simulink model "simModel2020"  (R2023b)
settings: Solver=ode4  StartTime=0  StopTime=360  FixedStep=0.01  RelTol=1e-3
values from neighbouring files (symbols this model uses):
  B747 =     [B747.mat]
undefined symbols (not defined in the file or in its folder): airport, APP, control, Curise, Earth, env, ft, m, navData, navParam, Newton, plotTrack, Raphson, s, TakeOff, WGS84
libraries: aerolibconvert2 x18, simulink x15, sharedtransform x4, aerolibfltsims x3, aerolibatmos2 x2, shared6dof x2, aerolibasang x2, dspsrcs4 x2, aerolibwind2 x2, aerolibanimutils x1, aerolibpropulsion2 x1, aerolibtransform2 x1
(part 3 of 6)

== system simModel2020/AutoPilot/InnerLoopAutopilot/Latitudinal Channel维度通道/Yaw Select/Filter1 ==
  x : Inport
  SW_x(k-1) : Inport  Port=2
  time : Inport  Port=3
  Constant : Constant  SampleTime=-1
  Data Type Conversion : DataTypeConversion  SaturateOnIntegerOverflow=off  RndMeth=Floor
  Detect Change : simulink/Logic and Bit Operations/Detect Change  vinit=0  OutDataTypeStr=boolean
  Gain : Gain  Gain=0.5
  Math Function : Math  SignedPower=on
  Product : Product
  Product1 : Product
  Subsystem : Subsystem
      mask Display: disp('S/H')
  Sum : Sum  Inputs=|+-
  Sum1 : Sum  Inputs=|++
  Sum2 : Sum  Inputs=+-|
  y : Outport
  wires:
  Product/1 -> Sum1/2
  SW_x(k-1)/1 -> Product/2
  Product1/1 -> Sum1/1
  x/1 -> Product1/1
  Sum1/1 -> Data Type Conversion/1
  time/1 -> Subsystem/1(In), Sum2/2
  Subsystem/1(" ") -> Sum2/1
  Sum2/1 -> Gain/1
  Gain/1 -> Math Function/1
  Math Function/1 -> Product/1, Sum/2
  Sum/1 -> Product1/2
  Data Type Conversion/1 -> y/1
  Constant/1 -> Sum/1, Detect Change/1
  Detect Change/1 -> Subsystem/Enable

== system simModel2020/AutoPilot/InnerLoopAutopilot/Longitudinal Channel经度通道/AutoThrottle/AT Mode = 0,Recycle ==
  dT(k-1) : Inport
  time : Inport  Port=2
  Action Port : ActionPort  InitializeStates=reset  ActionPortLabel=case [ 0 ]:
  Constant : Constant  Value=0.2
  Constant1 : Constant  Value=0
  Constant2 : Constant  Value=-0.2
  Filter1 : Subsystem
  Rate Limiter Dynamic with External IC and Autoreset for Change in IC : Subsystem
      mask Display:
      | plot([0.15 0.95],[.5 .5],[.5 .5],[0.05 0.95],0.05+0.9*[.2 .8],0.05+0.9*[0 1]);
      | port_label('output',1,'Y');
      | port_label('input',1,'up');
      | port_label('input',2,'u');
      | port_label('input',3,'Lo');
      | port_label('input',4,'IC');
  dT : Outport
  wires:
  dT(k-1)/1 -> Rate Limiter Dynamic with External IC and Autoreset for Change in IC/4(IC), Filter1/2(SW_x(k-1))
  Constant1/1 -> Filter1/1(x)
  time/1 -> Filter1/3(time)
  Rate Limiter Dynamic with External IC and Autoreset for Change in IC/1(Y) -> dT/1  "y"
  Filter1/1(y) -> Rate Limiter Dynamic with External IC and Autoreset for Change in IC/2(u)
  Constant/1 -> Rate Limiter Dynamic with External IC and Autoreset for Change in IC/1(up)
  Constant2/1 -> Rate Limiter Dynamic with External IC and Autoreset for Change in IC/3(lo)

== system simModel2020/AutoPilot/InnerLoopAutopilot/Longitudinal Channel经度通道/AutoThrottle/AT Mode = 2,MCP Speed ==
  <U_c> : Inport
  N1 : Inport  Port=2
  <ias> : Inport  Port=3
  dT(k-1) : Inport  Port=4
  time : Inport  Port=5
  Action Port : ActionPort  InitializeStates=reset  ActionPortLabel=case [ 2 ]:
  Add : Sum  Inputs=+-
  Filter1 : Subsystem
  Gain : Gain  Gain=10
  Mux : Mux  Inputs=2
  N1_Control : Subsystem
  Saturation1 : Saturate  UpperLimit=110  LowerLimit=0
  Scope : Scope
  Sum : Sum  Inputs=++|
  sat_integration : Subsystem
  dT : Outport
  wires:
  Gain/1 -> Sum/1
  dT(k-1)/1 -> Filter1/2(SW_x(k-1))
  Filter1/1(y) -> dT/1
  Add/1 -> sat_integration/1(err), Gain/1
  Sum/1 -> Saturation1/1
  N1_Control/1(dT) -> Filter1/1(x)
  N1/1 -> N1_Control/2(N1)
  Saturation1/1 -> N1_Control/1(N1_Cmd)
  sat_integration/1(int_err) -> Sum/2
  time/1 -> Filter1/3(time)
  <ias>/1 -> Mux/2, Add/2
  <U_c>/1 -> Mux/1, Add/1
  Mux/1 -> Scope/1

== system simModel2020/AutoPilot/InnerLoopAutopilot/Longitudinal Channel经度通道/AutoThrottle/AT Mode = 3,Throttle Control ==
  N1_Cmd : Inport
  N1 : Inport  Port=2
  dT(k-1) : Inport  Port=3
  time : Inport  Port=4
  Action Port : ActionPort  InitializeStates=reset  ActionPortLabel=case [ 3 ]:
  Add1 : Sum  Inputs=+-
  Derivative : Derivative
  Filter1 : Subsystem
  Gain : Gain  Gain=0.01
  Gain2 : Gain  Gain=0.02
  Integrator : Integrator
  Mux : Mux  Inputs=2
  Scope : Scope
  Sum : Sum  Inputs=++|
  Throttle Limit3 : Saturate  UpperLimit=0.2  LowerLimit=-0.2
      settings: AttributesFormatString="[%<LowerLimit>  %<UpperLimit>]"
  dT : Outport
  wires:
  Add1/1 -> Gain/1, Derivative/1
  dT(k-1)/1 -> Filter1/2(SW_x(k-1))
  Integrator/1 -> Filter1/1(x)
  Throttle Limit3/1 -> Integrator/1
  Derivative/1 -> Gain2/1
  Sum/1 -> Throttle Limit3/1
  Gain/1 -> Sum/2
  Gain2/1 -> Sum/1
  time/1 -> Filter1/3(time)
  N1/1 -> Mux/2, Add1/2
  N1_Cmd/1 -> Mux/1, Add1/1
  Mux/1 -> Scope/1
  Filter1/1(y) -> dT/1

== system simModel2020/AutoPilot/InnerLoopAutopilot/Longitudinal Channel经度通道/AutoThrottle/AT Mode = 5,Idle ==
  dT(k-1) : Inport
  time : Inport  Port=2
  Action Port : ActionPort  InitializeStates=reset  ActionPortLabel=case [ 5 ]:
  Constant : Constant  Value=0.2
  Constant1 : Constant  Value=B747.engine.Idle
  Constant2 : Constant  Value=-0.2
  Filter1 : Subsystem
  Rate Limiter Dynamic with External IC and Autoreset for Change in IC : Subsystem
      mask Display:
      | plot([0.15 0.95],[.5 .5],[.5 .5],[0.05 0.95],0.05+0.9*[.2 .8],0.05+0.9*[0 1]);
      | port_label('output',1,'Y');
      | port_label('input',1,'up');
      | port_label('input',2,'u');
      | port_label('input',3,'Lo');
      | port_label('input',4,'IC');
  dT : Outport
  wires:
  Constant/1 -> Rate Limiter Dynamic with External IC and Autoreset for Change in IC/1(up)
  Constant2/1 -> Rate Limiter Dynamic with External IC and Autoreset for Change in IC/3(lo)
  Rate Limiter Dynamic with External IC and Autoreset for Change in IC/1(Y) -> dT/1  "y"
  time/1 -> Filter1/3(time)
  dT(k-1)/1 -> Rate Limiter Dynamic with External IC and Autoreset for Change in IC/4(IC), Filter1/2(SW_x(k-1))
  Constant1/1 -> Filter1/1(x)
  Filter1/1(y) -> Rate Limiter Dynamic with External IC and Autoreset for Change in IC/2(u)

== system simModel2020/AutoPilot/InnerLoopAutopilot/Longitudinal Channel经度通道/AutoThrottle/Sample(1//z) ==
  <AT_Mode> : Inport
  x : Inport  Port=2
  Detect Change : Subsystem  mask(Detect Change){vinit=0, InputProcessing=Elements as channels (sample based), OutDataTypeStr=boolean}
      mask prompts: vinit "Simulink:masks:InitialCondition_MP"; InputProcessing "Simulink:masks:InputProcessing_MP"; OutDataTypeStr "Simulink:masks:OutputDataType_MP"
      mask help: Simulink:masks:DetectChange_MD
      mask init:
      | initDetectBlocks();
      mask TypeOptions InputProcessing: Simulink:masks:ColumnsAsChannelsFrameBased | Simulink:masks:ElementsAsChannelsSampleBased
      mask TypeOptions OutDataTypeStr: Simulink:masks:uint8 | Simulink:masks:boolean
      mask Display: fprintf('U ~= U/z')
  Sample and Hold : Subsystem  TreatAsAtomicUnit=on  mask(Sample and Hold){trig=Either edge, initCond=0, latchinput=off}
      mask prompts: trig "Trigger type:"; initCond "Initial condition:"; latchinput "Latch (buffer) input"
      mask help: Sample and hold the input signal. If Latch (buffer) input is selected, then this block produces the value of the input from the previous time step.
      mask init: same as simModel2020/AutoPilot/InnerLoopAutopilot/Latitudinal Channel维度通道/Sample(1//z)/Sample and Hold
      mask Help: eval('blocksethelp');
      mask TypeOptions trig: Rising edge | Falling edge | Either edge
      mask Display: disp('S/H')
  Unit Delay : UnitDelay  SampleTime=-1  HasFrameUpgradeWarning=on
  y : Outport
  wires:
  <AT_Mode>/1 -> Detect Change/1(U)
  Detect Change/1(Y) -> Sample and Hold/Trigger
  x/1 -> Unit Delay/1
  Unit Delay/1 -> Sample and Hold/1(In)
  Sample and Hold/1(" ") -> y/1

== system simModel2020/AutoPilot/InnerLoopAutopilot/Longitudinal Channel经度通道/PitchStyle/Altitude Hold ==
  h_Cmd : Inport
  h : Inport  Port=2
  Ve : Inport  Port=3
  Theta(k-1) : Inport  Port=4
  time : Inport  Port=5
  Action Port : ActionPort  InitializeStates=reset  ActionPortLabel=case [ 1 ]:
  Add2 : Sum  Inputs=+-
  Derivative : Derivative
  Filter1 : Subsystem
  Gain : Gain  Gain=0.2
  Gain1 : Gain  Gain=0.001
  Gain3 : Gain  Gain=0.035
  Integrator : Integrator  LimitOutput=on  UpperSaturationLimit=0.26  LowerSaturationLimit=-0.26
  Mux : Mux  Inputs=2
  Scope1 : Scope
  Selector : Selector  InputPortWidth=3  IndexOptions=Index vector (dialog)  Indices=[3]  OutputSizes=1
  Sum : Sum  Inputs=|+-
  Sum2 : Sum  Inputs=|++
  Theta_Cmd : Outport
  wires:
  Gain/1 -> Sum/1
  Ve/1 -> Selector/1
  Add2/1 -> Gain/1
  Selector/1 -> Sum/2
  Theta(k-1)/1 -> Filter1/2(SW_x(k-1))
  time/1 -> Filter1/3(time)
  Gain3/1 -> Sum2/2
  Derivative/1 -> Gain3/1
  Gain1/1 -> Sum2/1
  Sum2/1 -> Integrator/1
  Sum/1 -> Derivative/1, Gain1/1
  h_Cmd/1 -> Mux/1, Add2/1  "cmd_h"
  h/1 -> Mux/2, Add2/2  "theta"
  Integrator/1 -> Filter1/1(x)
  Mux/1 -> Scope1/1
  Filter1/1(y) -> Theta_Cmd/1

== system simModel2020/AutoPilot/InnerLoopAutopilot/Longitudinal Channel经度通道/PitchStyle/IAS_Control_dE ==
  IAS_Cmd : Inport
  <ias> : Inport  Port=2
  Theta(k-1) : Inport  Port=3
  time : Inport  Port=4
  Action Port : ActionPort  InitializeStates=reset  ActionPortLabel=case [ 0 ]:
  Add5 : Sum  Inputs=+-
  Derivative : Derivative
  Filter2 : Subsystem
  Gain : Gain  Gain=0.04
  Gain1 : Gain  Gain=-0.5
  Gain2 : Gain  Gain=0.005
  Integrator : Integrator  LimitOutput=on  UpperSaturationLimit=40  LowerSaturationLimit=-40
  Sum : Sum  Inputs=+++
  dE : Outport
  wires:
  Gain/1 -> Sum/1
  Add5/1 -> Integrator/1, Gain/1
  Integrator/1 -> Gain2/1
  <ias>/1 -> Derivative/1, Add5/2
  Gain2/1 -> Sum/2
  Theta(k-1)/1 -> Filter2/2(SW_x(k-1))
  Filter2/1(y) -> dE/1
  Sum/1 -> Filter2/1(x)
  IAS_Cmd/1 -> Add5/1
  Derivative/1 -> Gain1/1
  Gain1/1 -> Sum/3
  time/1 -> Filter2/3(time)

== system simModel2020/AutoPilot/InnerLoopAutopilot/Longitudinal Channel经度通道/PitchStyle/Pitch Control ==
  q : Inport
  Theta(k-1) : Inport  Port=2
  Pitch_Cmd : Inport  Port=3
  Euler : Inport  Port=4
  time : Inport  Port=5
  Action Port : ActionPort  InitializeStates=reset  ActionPortLabel=default:
  Add3 : Sum  Inputs=+-  OutDataTypeStr=single
  Add4 : Sum  Inputs=2  OutDataTypeStr=single
  Compute Feed Forward : Subsystem
  DEFFGain : Constant  Value=0  OutDataTypeStr=single
  Filter2 : Subsystem
  Gain : Gain  Gain=-10
  Gain1 : Gain  Gain=6
  Gain2 : Gain  Gain=57.3
  Mux : Mux  Inputs=2
  Scope : Scope
  Selector : Selector  InputPortWidth=3  IndexOptions=Index vector (dialog)  Indices=[1]  OutputSizes=1
  Selector2 : Selector  InputPortWidth=3  IndexOptions=Index vector (dialog)  Indices=[2]  OutputSizes=1
  Sum : Sum  Inputs=|++
  dE : Outport
  wires:
  Selector2/1 -> Add3/2, Mux/2  "theta"
  Sum/1 -> Add4/1
  Gain1/1 -> Sum/2
  Gain/1 -> Sum/1
  Euler/1 -> Selector/1, Selector2/1
  Selector/1 -> Compute Feed Forward/2(Roll)
  DEFFGain/1 -> Compute Feed Forward/1(dEFFGain)
  Add3/1 -> Gain/1
  Compute Feed Forward/1(FF) -> Add4/2
  Pitch_Cmd/1 -> Mux/1, Add3/1
  Theta(k-1)/1 -> Filter2/2(SW_x(k-1))
  q/1 -> Gain1/1
  time/1 -> Filter2/3(time)
  Mux/1 -> Gain2/1
  Add4/1 -> Filter2/1(x)
  Gain2/1 -> Scope/1
  Filter2/1(y) -> dE/1

== system simModel2020/AutoPilot/InnerLoopAutopilot/Longitudinal Channel经度通道/PitchStyle/Pitch Hold ==
  Theta : Inport
  Action Port : ActionPort  InitializeStates=reset  ActionPortLabel=case [ 3 ]:
  Theta_Cmd : Outport
  wires:
  Theta/1 -> Theta_Cmd/1

== system simModel2020/AutoPilot/InnerLoopAutopilot/Longitudinal Channel经度通道/PitchStyle/Rate Limiter Dynamic ==
  Test : Inport
  <Mode> : Inport  Port=2
  x : Inport  Port=3
  Constant1 : Constant  Value=5  OutDataTypeStr=double
  Constant2 : Constant  Value=-5  OutDataTypeStr=double
  Rate Limiter Dynamic with External IC and Autoreset for Change in IC1 : Subsystem
      mask Display:
      | plot([0.15 0.95],[.5 .5],[.5 .5],[0.05 0.95],0.05+0.9*[.2 .8],0.05+0.9*[0 1]);
      | port_label('output',1,'Y');
      | port_label('input',1,'up');
      | port_label('input',2,'u');
      | port_label('input',3,'Lo');
      | port_label('input',4,'IC');
  Sample(1/z) : Subsystem
  y : Outport
  wires:
  Sample(1/z)/1(y) -> Rate Limiter Dynamic with External IC and Autoreset for Change in IC1/4(IC)
  Constant1/1 -> Rate Limiter Dynamic with External IC and Autoreset for Change in IC1/1(up)
  x/1 -> Sample(1/z)/2(x)
  Rate Limiter Dynamic with External IC and Autoreset for Change in IC1/1(Y) -> y/1  "y"
  Constant2/1 -> Rate Limiter Dynamic with External IC and Autoreset for Change in IC1/3(lo)
  <Mode>/1 -> Sample(1/z)/1(<Test>)
  Test/1 -> Rate Limiter Dynamic with External IC and Autoreset for Change in IC1/2(u)

== system simModel2020/AutoPilot/InnerLoopAutopilot/Longitudinal Channel经度通道/PitchStyle/Rate Limiter Dynamic1 ==
  Test : Inport
  <Mode> : Inport  Port=2
  x : Inport  Port=3
  Constant1 : Constant  Value=15  OutDataTypeStr=double
  Constant2 : Constant  Value=-15  OutDataTypeStr=double
  Rate Limiter Dynamic with External IC and Autoreset for Change in IC : Subsystem
      mask Display:
      | plot([0.15 0.95],[.5 .5],[.5 .5],[0.05 0.95],0.05+0.9*[.2 .8],0.05+0.9*[0 1]);
      | port_label('output',1,'Y');
      | port_label('input',1,'up');
      | port_label('input',2,'u');
      | port_label('input',3,'Lo');
      | port_label('input',4,'IC');
  Sample(1/z) : Subsystem
  y : Outport
  wires:
  Sample(1/z)/1(y) -> Rate Limiter Dynamic with External IC and Autoreset for Change in IC/4(IC)
  Constant1/1 -> Rate Limiter Dynamic with External IC and Autoreset for Change in IC/1(up)
  Test/1 -> Rate Limiter Dynamic with External IC and Autoreset for Change in IC/2(u)
  x/1 -> Sample(1/z)/2(x)
  Rate Limiter Dynamic with External IC and Autoreset for Change in IC/1(Y) -> y/1  "y"
  Constant2/1 -> Rate Limiter Dynamic with External IC and Autoreset for Change in IC/3(lo)
  <Mode>/1 -> Sample(1/z)/1(<Test>)

== system simModel2020/AutoPilot/InnerLoopAutopilot/Longitudinal Channel经度通道/PitchStyle/Sample(1//z) ==
  <Mode> : Inport
  x : Inport  Port=2
  Detect Change : Subsystem  mask(Detect Change){vinit=0, InputProcessing=Elements as channels (sample based), OutDataTypeStr=boolean}
      mask prompts: vinit "Simulink:masks:InitialCondition_MP"; InputProcessing "Simulink:masks:InputProcessing_MP"; OutDataTypeStr "Simulink:masks:OutputDataType_MP"
      mask help: Simulink:masks:DetectChange_MD
      mask init:
      | initDetectBlocks();
      mask TypeOptions InputProcessing: Simulink:masks:ColumnsAsChannelsFrameBased | Simulink:masks:ElementsAsChannelsSampleBased
      mask TypeOptions OutDataTypeStr: Simulink:masks:uint8 | Simulink:masks:boolean
      mask Display: fprintf('U ~= U/z')
  Sample and Hold : Subsystem  TreatAsAtomicUnit=on  mask(Sample and Hold){trig=Either edge, initCond=0, latchinput=off}
      mask prompts: trig "Trigger type:"; initCond "Initial condition:"; latchinput "Latch (buffer) input"
      mask help: Sample and hold the input signal. If Latch (buffer) input is selected, then this block produces the value of the input from the previous time step.
      mask init: same as simModel2020/AutoPilot/InnerLoopAutopilot/Latitudinal Channel维度通道/Sample(1//z)/Sample and Hold
      mask Help: eval('blocksethelp');
      mask TypeOptions trig: Rising edge | Falling edge | Either edge
      mask Display: disp('S/H')
  Unit Delay : UnitDelay  SampleTime=-1  HasFrameUpgradeWarning=on
  y : Outport
  wires:
  <Mode>/1 -> Detect Change/1(U)
  Detect Change/1(Y) -> Sample and Hold/Trigger
  x/1 -> Unit Delay/1
  Unit Delay/1 -> Sample and Hold/1(In)
  Sample and Hold/1(" ") -> y/1

== system simModel2020/AutoPilot/InnerLoopAutopilot/Longitudinal Channel经度通道/PitchStyle/Sample(1//z)1 ==
  <Mode> : Inport
  x : Inport  Port=2
  Detect Change : Subsystem  mask(Detect Change){vinit=0, InputProcessing=Elements as channels (sample based), OutDataTypeStr=boolean}
      mask prompts: vinit "Simulink:masks:InitialCondition_MP"; InputProcessing "Simulink:masks:InputProcessing_MP"; OutDataTypeStr "Simulink:masks:OutputDataType_MP"
      mask help: Simulink:masks:DetectChange_MD
      mask init:
      | initDetectBlocks();
      mask TypeOptions InputProcessing: Simulink:masks:ColumnsAsChannelsFrameBased | Simulink:masks:ElementsAsChannelsSampleBased
      mask TypeOptions OutDataTypeStr: Simulink:masks:uint8 | Simulink:masks:boolean
      mask Display: fprintf('U ~= U/z')
  Sample and Hold : Subsystem  TreatAsAtomicUnit=on  mask(Sample and Hold){trig=Either edge, initCond=0, latchinput=off}
      mask prompts: trig "Trigger type:"; initCond "Initial condition:"; latchinput "Latch (buffer) input"
      mask help: Sample and hold the input signal. If Latch (buffer) input is selected, then this block produces the value of the input from the previous time step.
      mask init: same as simModel2020/AutoPilot/InnerLoopAutopilot/Latitudinal Channel维度通道/Sample(1//z)/Sample and Hold
      mask Help: eval('blocksethelp');
      mask TypeOptions trig: Rising edge | Falling edge | Either edge
      mask Display: disp('S/H')
  Unit Delay : UnitDelay  SampleTime=-1  HasFrameUpgradeWarning=on
  y : Outport
  wires:
  Sample and Hold/1(" ") -> y/1
  Unit Delay/1 -> Sample and Hold/1(In)
  x/1 -> Unit Delay/1
  Detect Change/1(Y) -> Sample and Hold/Trigger
  <Mode>/1 -> Detect Change/1(U)

== system simModel2020/AutoPilot/InnerLoopAutopilot/Longitudinal Channel经度通道/PitchStyle/Vtertical Speed Control ==
  Theta(k-1) : Inport
  Ve : Inport  Port=2
  VertSpeedCmd : Inport  Port=3
  time : Inport  Port=4
  Action Port : ActionPort  InitializeStates=reset  ActionPortLabel=case [ 2 ]:
  Add1 : Sum  Inputs=+-  OutDataTypeStr=single
  Data Type Conversion : DataTypeConversion  SaturateOnIntegerOverflow=off  RndMeth=Floor
  Derivative : Derivative
  Filter1 : Subsystem
  Gain3 : Gain  Gain=0.002
  Gain4 : Gain  Gain=0.01
  Integrator : Integrator  LimitOutput=on  UpperSaturationLimit=0.26  LowerSaturationLimit=-0.26
  Mux : Mux  Inputs=2
  Scope1 : Scope
  Selector4 : Selector  InputPortWidth=3  IndexOptions=Index vector (dialog)  Indices=[3]  OutputSizes=1
  Sum2 : Sum  Inputs=|++
  Theta_Cmd : Outport
  wires:
  VertSpeedCmd/1 -> Add1/1, Mux/1  "cmd_h"
  Ve/1 -> Selector4/1
  Theta(k-1)/1 -> Filter1/2(SW_x(k-1))
  time/1 -> Filter1/3(time)
  Gain3/1 -> Sum2/1
  Derivative/1 -> Gain4/1
  Add1/1 -> Data Type Conversion/1
  Sum2/1 -> Integrator/1
  Gain4/1 -> Sum2/2
  Data Type Conversion/1 -> Derivative/1, Gain3/1
  Selector4/1 -> Mux/2, Add1/2  "dh"
  Integrator/1 -> Filter1/1(x)
  Mux/1 -> Scope1/1
  Filter1/1(y) -> Theta_Cmd/1

== system simModel2020/PlantModel/B747 Dynamics动力学参数计算/6DOF Equations of Motion运动学方程/[0, pi] Wrap Around/Compare To Zero ==
  u : Inport
  Compare : RelationalOperator  OutDataTypeStr=fixdt(0, 8)  ZeroCross=off
  Constant : Constant  DisableCoverage=on  Value=0  OutDataTypeStr=Inherit: Inherit via back propagation  PreserveConstantTs=on
  y : Outport
  wires:
  Constant/1 -> Compare/2
  u/1 -> Compare/1
  Compare/1 -> y/1

== system simModel2020/PlantModel/B747 Dynamics动力学参数计算/6DOF Equations of Motion运动学方程/[0, pi] Wrap Around/Negative Yaw ==
  yaw : Inport
  Enable : EnablePort
  Abs : Abs  SaturateOnIntegerOverflow=off
  Constant1 : Constant  Value=2*pi
      settings: AttributesFormatString=%<Value>
  Constant2 : Constant  Value=2*pi
      settings: AttributesFormatString=%<Value>
  Math Function : Math  Operator=mod  SignedPower=on
  Sum : Sum  Inputs=|-+
  yaw_wr : Outport
  wires:
  Sum/1 -> yaw_wr/1
  Constant2/1 -> Sum/2
  Abs/1 -> Math Function/1
  Math Function/1 -> Sum/1
  Constant1/1 -> Math Function/2
  yaw/1 -> Abs/1

== system simModel2020/PlantModel/B747 Dynamics动力学参数计算/6DOF Equations of Motion运动学方程/[0, pi] Wrap Around/Positive Yaw ==
  yaw : Inport
  Enable : EnablePort
  Constant1 : Constant  Value=2*pi
      settings: AttributesFormatString=%<Value>
  Math Function : Math  Operator=mod  SignedPower=on
  yaw_wr : Outport
  wires:
  Math Function/1 -> yaw_wr/1
  Constant1/1 -> Math Function/2
  yaw/1 -> Math Function/1

== system simModel2020/PlantModel/B747 Dynamics动力学参数计算/Forces and Moments动力学计算/Compute Air Data迎角侧滑角计算/Dynamic Pressure动压 ==
  Velocity : Inport
  Air Density : Inport  Port=2
  1/2rhoV^2 : Gain  Gain=1/2  SaturateOnIntegerOverflow=on  OutDataTypeStr=Inherit: Same as input  ParamDataTypeStr=Inherit: Same as input
  Product2 : Product  InputSameDT=on  SaturateOnIntegerOverflow=on  OutDataTypeStr=Inherit: Same as first input
  dot : Subsystem
  qbar : Outport  InitialOutput=0
  wires:
  1/2rhoV^2/1 -> qbar/1
  Product2/1 -> 1/2rhoV^2/1
  Air Density/1 -> Product2/2
  dot/1(dot) -> Product2/1
  Velocity/1 -> dot/1(V)

== system simModel2020/PlantModel/B747 Dynamics动力学参数计算/Forces and Moments动力学计算/Compute Body Frame Forces and Moments气动力和力矩/Rotate FM to body frame ==
  FM_w : Inport
  alpha_beta : Inport  Port=2
  Forces : Selector  InputPortWidth=6  IndexOptions=Index vector (dialog)  Indices=[1 2 3]  OutputSizes=[(-2)]
  Moments : Selector  InputPortWidth=6  IndexOptions=Index vector (dialog)  Indices=[4 5 6]  OutputSizes=[(-2)]
  Rotate Forces : Subsystem
  Rotate Moments : Subsystem
  F_b : Outport
  M_b : Outport  Port=2
  wires:
  alpha_beta/1 -> Rotate Forces/2(alpha_beta), Rotate Moments/1(alpha_beta)
  Moments/1 -> Rotate Moments/2(M_w)
  FM_w/1 -> Moments/1, Forces/1
  Forces/1 -> Rotate Forces/1(F_w)
  Rotate Moments/1(M_b) -> M_b/1
  Rotate Forces/1(F_b) -> F_b/1

== system simModel2020/PlantModel/B747 Dynamics动力学参数计算/Forces and Moments动力学计算/Compute Body Frame Forces and Moments气动力和力矩/Wind frame F& M 气动力计算 ==
  Airdata : Inport
  CtrlSurfaces : Inport  Port=2
  p,q,r : Inport  Port=3
  Deviation On : Inport  Port=4
  Bus Creator1 : BusCreator  Inputs=2
  Bus Selector1 : BusSelector  OutputSignals=dA,dR
  Bus Selector2 : BusSelector  OutputSignals=dE,dF
  Bus Selector6 : BusSelector  OutputSignals=beta,airpseed
  Bus Selector7 : BusSelector  OutputSignals=alpha,airpseed
  Get Forces and Moments : Subsystem
  Lateral Channel : Subsystem
  Longitudinal Channel : Subsystem
  FM_w : Outport  PortDimensions=6
  wires:
  Get Forces and Moments/1(FM_w) -> FM_w/1
  Bus Creator1/1 -> Get Forces and Moments/2(AeroCoeffs)
  Bus Selector7/2 -> Longitudinal Channel/2(Airpseed)  "<airpseed>"
  Bus Selector7/1 -> Longitudinal Channel/1(alpha)  "<alpha>"
  Bus Selector6/2 -> Lateral Channel/2(Airspeed)  "<airpseed>"
  Bus Selector6/1 -> Lateral Channel/1(beta)  "<beta>"
  Airdata/1 -> Bus Selector7/1, Get Forces and Moments/1(Airdata), Bus Selector6/1
  Bus Selector2/2 -> Longitudinal Channel/4(dF)  "<dF>"
  Bus Selector2/1 -> Longitudinal Channel/3(dE)  "<dE>"
  Bus Selector1/2 -> Lateral Channel/4(dR)  "<dR>"
  Bus Selector1/1 -> Lateral Channel/3(dA)  "<dA>"
  CtrlSurfaces/1 -> Bus Selector2/1, Bus Selector1/1
  p,q,r/1 -> Longitudinal Channel/5(p,q,r), Lateral Channel/5(p,q,r)
  Lateral Channel/1(Lateral) -> Bus Creator1/1
  Longitudinal Channel/1(Longitudinal) -> Bus Creator1/2
  Deviation On/1 -> Longitudinal Channel/6(Deviation On), Lateral Channel/6(Deviation On)

== system simModel2020/PlantModel/B747 Dynamics动力学参数计算/Forces and Moments动力学计算/Engine Model/ Turbofan Engine System ==
  note: T_sta
  note: C_T
  note: PLA
  note: 1燃油速率
      | 2发动机推力
      | 3低压转子转速
  Throttle_cmd : Inport
  Mach : Inport  Port=2
  Altitude : Inport  Port=3
  Calculate delta and theta : aerolibpropulsion2/Turbofan Engine System/Calculate delta and theta  SystemSampleTime=-1  VariantActivationTime=update diagram  AllowFlexibleInterface=on  Latency=0  AutoFrameSizeCalculation=off
  Display : Display
  Fmax : Constant  Value=Fmax
  Gain3 : Gain  Gain=Nt  SaturateOnIntegerOverflow=on  OutDataTypeStr=Inherit: Same as input  ParamDataTypeStr=Inherit: Same as input
  Length Conversion : aerolibconvert2/Length Conversion  IU=m  OU=ft
  N1 caculation 包含大气参数计算 : Subsystem
  Non-dimensional C_SFC(Thrust,Mach) : Lookup_n-D  BreakpointsForDimension1=[0.0:0.04:1.0]  BreakpointsForDimension2=[0:.1:1]  IndexSearchMethod=Linear search  BeginIndexSearchUsingPreviousIndexResult=on  Table=C_SFC  ExtrapMethod=Clip  DiagnosticForOutOfRangeInput=Warning
      mask init:
      | C_SFC=[2.06 2.16 2.31 2.83 2.97 3.11 3.35 3.59 3.62 3.66 3.7;
      |     1.8437 1.9437 2.0937 2.5565 2.6965 2.8365 3.0597 3.2997 3.3297 3.3697 3.4097;
      |     1.6618 1.7618 1.9118 2.3228 2.4628 2.6028 2.8092 3.0492 3.0792 3.1192 3.1592;
      |     1.5104 1.6104 1.7604 2.1248 2.2648 2.4048 2.5948 2.8348 2.8648 2.9048 2.9448;
      |     1.3861 1.4861 1.6361 1.9587 2.0987 2.2387 2.413 2.653 2.683 2.723 2.763;
      |     1.2854 1.3854 1.5354 1.8206 1.9606 2.1006 2.2603 2.5003 2.5303 2.5703 2.6103;
      |     1.2052 1.3052 1.4552 1.7074 1.8474 1.9874 2.1335 2.3735 2.4035 2.4435 2.4835;
      |     1.1425 1.2425 1.3925 1.6156 1.7556 1.8956 2.0295 2.2695 2.2995 2.3395 2.3795;
      |     1.0948 1.1948 1.3448 1.5425 1.6825 1.8225 1.9455 2.1855 2.2155 2.2555 2.2955;
      |     1.0594 1.1594 1.3094 1.4851 1.6251 1.7651 1.8789 2.1189 2.1489 2.1889 2.2289;
      |     1.0342 1.1342 1.2842 1.441 1.581 1.721 1.8271 2.0671 2.0971 2.1371 2.1771;
      |     1.017 1.117 1.267 1.4079 1.5479 1.6879 1.7879 2.0279 2.0579 2.0979 2.1379;
      |     1.0061 1.1061 1.2561 1.3837 1.5237 1.6637 1.7592 1.9992 2.0292 2.0692 2.1092;
      |     0.9999 1.0999 1.2499 1.3666 1.5066 1.6466 1.739 1.979 2.009 2.049 2.089;
      |     0.9969 1.0969 1.2469 1.3548 1.4948 1.6348 1.7256 1.9656 1.9956 2.0356 2.0756;
      |     0.9959 1.0959 1.2459 1.347 1.487 1.627 1.7176 1.9576 1.9876 2.0276 2.0676;
      |     0.9961 1.0961 1.2461 1.3421 1.4821 1.6221 1.7134 1.9534 1.9834 2.0234 2.0634;
      |     0.9968 1.0968 1.2468 1.339 1.479 1.619 1.712 1.952 1.982 2.022 2.062;
      |     0.9972 1.0972 1.2472 1.337 1.477 1.617 1.7123 1.9523 1.9823 2.0223 2.0623;
      |     0.9973 1.0973 1.2473 1.3357 1.4757 1.6157 1.7136 1.9536 1.9836 2.0236 2.0636;
      |     0.9969 1.0969 1.2469 1.3346 1.4746 1.6146 1.7152 1.9552 1.9852 2.0252 2.0652;
      |     0.9961 1.0961 1.2461 1.3339 1.4739 1.6139 1.7168 1.9568 1.9868 2.0268 2.0668;
      |     0.9954 1.0954 1.2454 1.3335 1.4735 1.6135 1.718 1.958 1.988 2.028 2.068;
      |     0.9952 1.0952 1.2452 1.334 1.474 1.614 1.7188 1.9588 1.9888 2.0288 2.0688;
      |     0.9964	1.0964 1.2464 1.3359 1.4759 1.6159 1.7194 1.9594 1.9894 2.0294 2.0694;
      |     1	1.1 1.25 1.34 1.48 1.62 1.72 1.96 1.99 2.03 2.07];
      settings: InputPortMap=u0,u1
  Non-dimensional C_Thrust(Throttle,Mach) : Lookup_n-D  BreakpointsForDimension1=[0 1]  BreakpointsForDimension2=[0:.1:1]  BreakpointsForDimension3=[0 1]  IndexSearchMethod=Linear search  BeginIndexSearchUsingPreviousIndexResult=on  Table=Non_dimensional_Thrust  ExtrapMethod=Clip  DiagnosticForOutOfRangeInput=Warning
      mask init:
      | Non_dimensional_Thrust=[0 0 0 0 0 0 0 0 0 0 0; 
      |     1 0.92 0.84 0.76 0.68 0.6 0.58 0.56 0.54 0.52 0.5];
      settings: InputPortMap=u0,u1
  Product4 : Product  Inputs=**/**  InputSameDT=on  SaturateOnIntegerOverflow=on  OutDataTypeStr=Inherit: Same as first input
  SFC : Constant  Value=SFC
  Subsystem : Subsystem
  T_tgt : Product  Inputs=3  InputSameDT=on  SaturateOnIntegerOverflow=on  OutDataTypeStr=Inherit: Same as first input
  Transfer function : Subsystem
  hr2sec : Constant  Value=3600
  Thrust(N) : Outport
  Fuel flow(kg/s) : Outport  Port=2
  N1 : Outport  Port=3
  wires:
  SFC/1 -> Product4/2
  hr2sec/1 -> Product4/3
  Gain3/1 -> Thrust(N)/1
  Altitude/1 -> N1 caculation 包含大气参数计算/3(Altitude), Length Conversion/1
  Length Conversion/1 -> Calculate delta and theta/1
  Product4/1 -> Fuel flow(kg/s)/1
  Non-dimensional C_Thrust(Throttle,Mach)/1 -> Non-dimensional C_SFC(Thrust,Mach)/1, T_tgt/2
  Fmax/1 -> T_tgt/3
  Calculate delta and theta/1 -> N1 caculation 包含大气参数计算/1(sqrt(theta)), Subsystem/2(sqrt(theta)), Product4/4
  Non-dimensional C_SFC(Thrust,Mach)/1 -> Product4/1
  Calculate delta and theta/2 -> Subsystem/3(delta), T_tgt/1
  Transfer function/1(T_out) -> Gain3/1, Product4/5, Subsystem/1(thrust)
  Subsystem/1(tau) -> Transfer function/1(tau)
  T_tgt/1 -> Transfer function/2(T_tgt)
  Throttle_cmd/1 -> N1 caculation 包含大气参数计算/2(Throttle_cmd), Non-dimensional C_Thrust(Throttle,Mach)/1
  Mach/1 -> Non-dimensional C_SFC(Thrust,Mach)/2, N1 caculation 包含大气参数计算/4(Mach), Non-dimensional C_Thrust(Throttle,Mach)/2, Calculate delta and theta/2
  N1 caculation 包含大气参数计算/1(N1(%)) -> Display/1, N1/1

== system simModel2020/PlantModel/B747 Dynamics动力学参数计算/Forces and Moments动力学计算/Rotate Vw/RL2B ==
  Euler : Inport
  Rotation Angles to Direction Cosine Matrix1 : sharedtransform/Rotation Angles to Direction Cosine Matrix  rotationOrder=ZYX  aMode=aMode
  Selector : Selector  InputPortWidth=3  IndexOptions=Index vector (dialog)  Indices=[3 2 1]  OutputSizes=1
  RL2B : Outport
  wires:
  Rotation Angles to Direction Cosine Matrix1/1 -> RL2B/1
  Euler/1 -> Selector/1
  Selector/1 -> Rotation Angles to Direction Cosine Matrix1/1

== system simModel2020/PlantModel/B747 Dynamics动力学参数计算/Forces and Moments动力学计算/Rotate g to Body Frame/RL2B ==
  Euler : Inport
  Rotation Angles to Direction Cosine Matrix1 : sharedtransform/Rotation Angles to Direction Cosine Matrix  rotationOrder=ZYX  aMode=aMode
  Selector : Selector  InputPortWidth=3  IndexOptions=Index vector (dialog)  Indices=[3 2 1]  OutputSizes=1
  RL2B : Outport
  wires:
  Rotation Angles to Direction Cosine Matrix1/1 -> RL2B/1
  Euler/1 -> Selector/1
  Selector/1 -> Rotation Angles to Direction Cosine Matrix1/1

== system simModel2020/PlantModel/B747 Dynamics动力学参数计算/Forces and Moments动力学计算/Touch the Ground Detection/RL2B ==
  Euler : Inport
  Rotation Angles to Direction Cosine Matrix1 : sharedtransform/Rotation Angles to Direction Cosine Matrix  rotationOrder=ZYX  aMode=aMode
  Selector : Selector  InputPortWidth=3  IndexOptions=Index vector (dialog)  Indices=[3 2 1]  OutputSizes=1
  RL2B : Outport
  wires:
  Rotation Angles to Direction Cosine Matrix1/1 -> RL2B/1
  Euler/1 -> Selector/1
  Selector/1 -> Rotation Angles to Direction Cosine Matrix1/1

== system simModel2020/PlantModel/B747 Dynamics动力学参数计算/Forces and Moments动力学计算/Touch the Ground Detection/dot ==
  Vb : Inport
  Demux1 : Demux  Outputs=3
  Product : Product  RndMeth=Zero
  Product1 : Product  RndMeth=Zero
  Product2 : Product  RndMeth=Zero
  Sum : Sum  Inputs=+++
  dot : Outport
  wires:
  Product2/1 -> Sum/3
  Demux1/3 -> Product2/2, Product2/1
  Product/1 -> Sum/1
  Product1/1 -> Sum/2
  Sum/1 -> dot/1
  Vb/1 -> Demux1/1
  Demux1/1 -> Product/2, Product/1
  Demux1/2 -> Product1/1, Product1/2

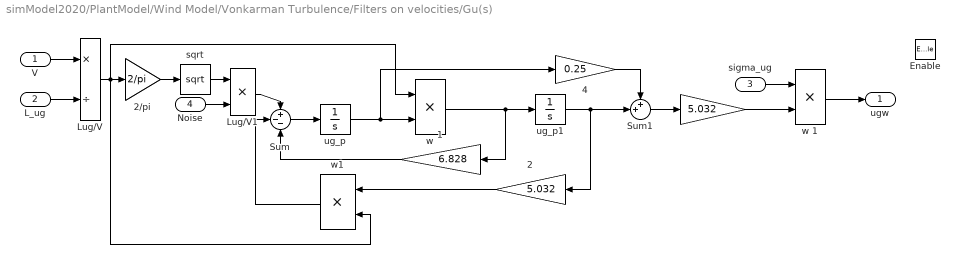
== system simModel2020/PlantModel/Wind Model/Vonkarman Turbulence/Filters on velocities/Gu(s) ==
  V : Inport
  L_ug : Inport  Port=2
  sigma_ug : Inport  Port=3
  Noise : Inport  Port=4
  Enable : EnablePort
  " " : Gain  Gain=5.032  SaturateOnIntegerOverflow=on  OutDataTypeStr=Inherit: Same as input  ParamDataTypeStr=Inherit: Same as input
  " 1" : Gain  Gain=6.828  SaturateOnIntegerOverflow=on  OutDataTypeStr=Inherit: Same as input  ParamDataTypeStr=Inherit: Same as input
  " 2" : Gain  Gain=5.032  SaturateOnIntegerOverflow=on  OutDataTypeStr=Inherit: Same as input  ParamDataTypeStr=Inherit: Same as input
  2/pi : Gain  Gain=2/pi  SaturateOnIntegerOverflow=on  OutDataTypeStr=Inherit: Same as input  ParamDataTypeStr=Inherit: Same as input
  4 : Gain  Gain=0.25  SaturateOnIntegerOverflow=on  OutDataTypeStr=Inherit: Same as input  ParamDataTypeStr=Inherit: Same as input
  Lug/V : Product  Inputs=*/  InputSameDT=on  SaturateOnIntegerOverflow=on  OutDataTypeStr=Inherit: Same as first input
  Lug/V1 : Product  InputSameDT=on  SaturateOnIntegerOverflow=on  OutDataTypeStr=Inherit: Same as first input
  Sum : Sum  Inputs=+--  InputSameDT=on  SaturateOnIntegerOverflow=on  OutDataTypeStr=Inherit: Same as first input
  Sum1 : Sum  Inputs=++|  InputSameDT=on  SaturateOnIntegerOverflow=on  OutDataTypeStr=Inherit: Same as first input
  sqrt : Sqrt  AlgorithmType=Newton-Raphson
  ug_p : Integrator  InitialCondition=1
  ug_p1 : Integrator
  w : Product  InputSameDT=on  SaturateOnIntegerOverflow=on  OutDataTypeStr=Inherit: Same as first input
  w 1 : Product  InputSameDT=on  SaturateOnIntegerOverflow=on  OutDataTypeStr=Inherit: Same as first input
  w1 : Product  InputSameDT=on  SaturateOnIntegerOverflow=on  OutDataTypeStr=Inherit: Same as first input
  ugw : Outport  OutputWhenDisabled=reset  InitialOutput=0
  wires:
  2/pi/1 -> sqrt/1
  ug_p/1 -> 4/1, w/2
  w1/1 -> Sum/2
  V/1 -> Lug/V/1
  ug_p1/1 -> " 2"/1, Sum1/2
  w 1/1 -> ugw/1
  Lug/V/1 -> 2/pi/1, w1/2, w/1
  4/1 -> Sum1/1
  L_ug/1 -> Lug/V/2
  w/1 -> ug_p1/1, " 1"/1
  Sum1/1 -> " "/1
  " "/1 -> w 1/2
  " 2"/1 -> w1/1
  Lug/V1/1 -> Sum/1
  " 1"/1 -> Sum/3
  Sum/1 -> ug_p/1
  Noise/1 -> Lug/V1/2
  sqrt/1 -> Lug/V1/1
  sigma_ug/1 -> w 1/1

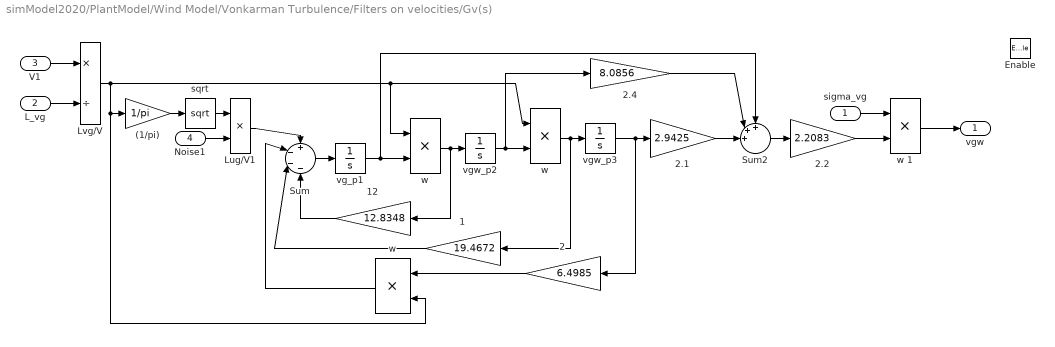
== system simModel2020/PlantModel/Wind Model/Vonkarman Turbulence/Filters on velocities/Gv(s) ==
  sigma_vg : Inport
  L_vg : Inport  Port=2
  V1 : Inport  Port=3
  Noise1 : Inport  Port=4
  Enable : EnablePort
  " w" : Product  InputSameDT=on  SaturateOnIntegerOverflow=on  OutDataTypeStr=Inherit: Same as first input
  (1/pi) : Gain  Gain=1/pi  SaturateOnIntegerOverflow=on  OutDataTypeStr=Inherit: Same as input  ParamDataTypeStr=Inherit: Same as input
  1 : Gain  Gain=19.4672  SaturateOnIntegerOverflow=on  OutDataTypeStr=Inherit: Same as input  ParamDataTypeStr=Inherit: Same as input
  12 : Gain  Gain=12.8348  SaturateOnIntegerOverflow=on  OutDataTypeStr=Inherit: Same as input  ParamDataTypeStr=Inherit: Same as input
  2 : Gain  Gain=6.4985  SaturateOnIntegerOverflow=on  OutDataTypeStr=Inherit: Same as input  ParamDataTypeStr=Inherit: Same as input
  2.1 : Gain  Gain=2.9425  SaturateOnIntegerOverflow=on  OutDataTypeStr=Inherit: Same as input  ParamDataTypeStr=Inherit: Same as input
  2.2 : Gain  Gain=2.2083  SaturateOnIntegerOverflow=on  OutDataTypeStr=Inherit: Same as input  ParamDataTypeStr=Inherit: Same as input
  2.4 : Gain  Gain=8.0856  SaturateOnIntegerOverflow=on  OutDataTypeStr=Inherit: Same as input  ParamDataTypeStr=Inherit: Same as input
  Lug/V1 : Product  InputSameDT=on  SaturateOnIntegerOverflow=on  OutDataTypeStr=Inherit: Same as first input
  Lvg/V : Product  Inputs=*/  InputSameDT=on  SaturateOnIntegerOverflow=on  OutDataTypeStr=Inherit: Same as first input
  Sum : Sum  Inputs=+---  InputSameDT=on  SaturateOnIntegerOverflow=on  OutDataTypeStr=Inherit: Same as first input
  Sum2 : Sum  Inputs=+++||  InputSameDT=on  SaturateOnIntegerOverflow=on  OutDataTypeStr=Inherit: Same as first input
  sqrt : Sqrt  AlgorithmType=Newton-Raphson
  vg_p1 : Integrator
  vgw_p2 : Integrator
  vgw_p3 : Integrator
  w : Product  InputSameDT=on  SaturateOnIntegerOverflow=on  OutDataTypeStr=Inherit: Same as first input
  "w " : Product  InputSameDT=on  SaturateOnIntegerOverflow=on  OutDataTypeStr=Inherit: Same as first input
  w 1 : Product  InputSameDT=on  SaturateOnIntegerOverflow=on  OutDataTypeStr=Inherit: Same as first input
  vgw : Outport  OutputWhenDisabled=reset  InitialOutput=0
  wires:
  sqrt/1 -> Lug/V1/1
  Lug/V1/1 -> Sum/1
  Lvg/V/1 -> " w"/2, (1/pi)/1, w/1, "w "/1
  vgw_p2/1 -> 2.4/1, w/2
  "w "/1 -> vgw_p2/1, 12/1
  sigma_vg/1 -> w 1/1
  L_vg/1 -> Lvg/V/2
  12/1 -> Sum/4
  (1/pi)/1 -> sqrt/1
  " w"/1 -> Sum/2
  Sum/1 -> vg_p1/1
  2.1/1 -> Sum2/3
  Noise1/1 -> Lug/V1/2
  Sum2/1 -> 2.2/1
  vg_p1/1 -> Sum2/1, "w "/2
  2.4/1 -> Sum2/2
  2.2/1 -> w 1/2
  w/1 -> vgw_p3/1, 1/1
  w 1/1 -> vgw/1
  2/1 -> " w"/1
  vgw_p3/1 -> 2.1/1, 2/1
  V1/1 -> Lvg/V/1
  1/1 -> Sum/3

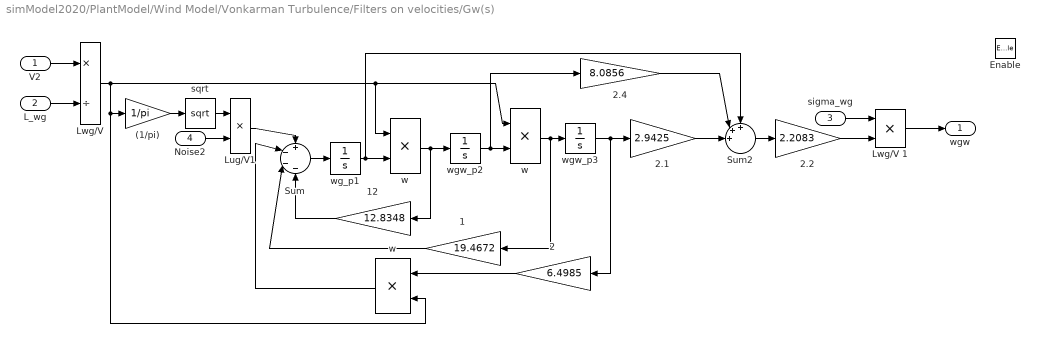
== system simModel2020/PlantModel/Wind Model/Vonkarman Turbulence/Filters on velocities/Gw(s) ==
  V2 : Inport
  L_wg : Inport  Port=2
  sigma_wg : Inport  Port=3
  Noise2 : Inport  Port=4
  Enable : EnablePort
  " w" : Product  InputSameDT=on  SaturateOnIntegerOverflow=on  OutDataTypeStr=Inherit: Same as first input
  (1/pi) : Gain  Gain=1/pi  SaturateOnIntegerOverflow=on  OutDataTypeStr=Inherit: Same as input  ParamDataTypeStr=Inherit: Same as input
  1 : Gain  Gain=19.4672  SaturateOnIntegerOverflow=on  OutDataTypeStr=Inherit: Same as input  ParamDataTypeStr=Inherit: Same as input
  12 : Gain  Gain=12.8348  SaturateOnIntegerOverflow=on  OutDataTypeStr=Inherit: Same as input  ParamDataTypeStr=Inherit: Same as input
  2 : Gain  Gain=6.4985  SaturateOnIntegerOverflow=on  OutDataTypeStr=Inherit: Same as input  ParamDataTypeStr=Inherit: Same as input
  2.1 : Gain  Gain=2.9425  SaturateOnIntegerOverflow=on  OutDataTypeStr=Inherit: Same as input  ParamDataTypeStr=Inherit: Same as input
  2.2 : Gain  Gain=2.2083  SaturateOnIntegerOverflow=on  OutDataTypeStr=Inherit: Same as input  ParamDataTypeStr=Inherit: Same as input
  2.4 : Gain  Gain=8.0856  SaturateOnIntegerOverflow=on  OutDataTypeStr=Inherit: Same as input  ParamDataTypeStr=Inherit: Same as input
  Lug/V1 : Product  InputSameDT=on  SaturateOnIntegerOverflow=on  OutDataTypeStr=Inherit: Same as first input
  Lwg/V : Product  Inputs=*/  InputSameDT=on  SaturateOnIntegerOverflow=on  OutDataTypeStr=Inherit: Same as first input
  Lwg/V 1 : Product  InputSameDT=on  SaturateOnIntegerOverflow=on  OutDataTypeStr=Inherit: Same as first input
  Sum : Sum  Inputs=+---  InputSameDT=on  SaturateOnIntegerOverflow=on  OutDataTypeStr=Inherit: Same as first input
  Sum2 : Sum  Inputs=+++||  InputSameDT=on  SaturateOnIntegerOverflow=on  OutDataTypeStr=Inherit: Same as first input
  sqrt : Sqrt  AlgorithmType=Newton-Raphson
  w : Product  InputSameDT=on  SaturateOnIntegerOverflow=on  OutDataTypeStr=Inherit: Same as first input
  "w " : Product  InputSameDT=on  SaturateOnIntegerOverflow=on  OutDataTypeStr=Inherit: Same as first input
  wg_p1 : Integrator  UpperSaturationLimit=10  LowerSaturationLimit=-10
  wgw_p2 : Integrator
  wgw_p3 : Integrator
  wgw : Outport  OutputWhenDisabled=reset  InitialOutput=0
  wires:
  2.2/1 -> Lwg/V 1/2
  Lug/V1/1 -> Sum/1
  Sum2/1 -> 2.2/1
  wgw_p2/1 -> 2.4/1, w/2
  L_wg/1 -> Lwg/V/2
  sigma_wg/1 -> Lwg/V 1/1
  2.1/1 -> Sum2/3
  "w "/1 -> wgw_p2/1, 12/1
  2.4/1 -> Sum2/2
  Lwg/V/1 -> " w"/2, (1/pi)/1, w/1, "w "/1
  wg_p1/1 -> Sum2/1, "w "/2
  Lwg/V 1/1 -> wgw/1
  w/1 -> wgw_p3/1, 1/1
  (1/pi)/1 -> sqrt/1
  sqrt/1 -> Lug/V1/1
  wgw_p3/1 -> 2.1/1, 2/1
  1/1 -> Sum/3
  Noise2/1 -> Lug/V1/2
  V2/1 -> Lwg/V/1
  2/1 -> " w"/1
  " w"/1 -> Sum/2
  12/1 -> Sum/4
  Sum/1 -> wg_p1/1

== system simModel2020/PlantModel/Wind Model/Vonkarman Turbulence/Turbulence scale lengths/Low altitude scale length ==
  h : Inport
  Limit Function 10ft to 1000ft : Saturate  UpperLimit=max_height_low  LowerLimit=10
  Low Altitude Scale Length : Fcn  Expr=u(1)/(0.177+0.000823*u(1))^1.2
  L_ug L_vg : Outport  InitialOutput=0
  L_wg : Outport  Port=2  InitialOutput=0
  wires:
  h/1 -> Limit Function 10ft to 1000ft/1
  Limit Function 10ft to 1000ft/1 -> L_wg/1, Low Altitude Scale Length/1
  Low Altitude Scale Length/1 -> L_ug L_vg/1

== system simModel2020/PlantModel/Wind Model/Vonkarman Turbulence/Turbulence scale lengths/Subsystem ==
  Length Conversion : aerolibconvert2/Length Conversion  IU=ft  OU=m
  Medium/High Altitude : Constant  Value=L_high  OutDataTypeStr=Inherit: Inherit via back propagation
  L_ug L_vg L_wg : Outport  InitialOutput=0
  wires:
  Length Conversion/1 -> L_ug L_vg L_wg/1
  Medium/High Altitude/1 -> Length Conversion/1

== system simModel2020/AutoPilot/InnerLoopAutopilot/Latitudinal Channel维度通道/Lateral Correction/Filter1/Subsystem ==
  In : Inport
  Enable : EnablePort  StatesWhenEnabling=reset
  " " : Outport  InitialOutput=0
  wires:
  In/1 -> " "/1

== system simModel2020/AutoPilot/InnerLoopAutopilot/Latitudinal Channel维度通道/Roll Control/Filter1/Subsystem ==
  In : Inport
  Enable : EnablePort  StatesWhenEnabling=reset
  " " : Outport  InitialOutput=0
  wires:
  In/1 -> " "/1

== system simModel2020/AutoPilot/InnerLoopAutopilot/Latitudinal Channel维度通道/Yaw Select/Filter1/Subsystem ==
  In : Inport
  Enable : EnablePort  StatesWhenEnabling=reset
  " " : Outport  InitialOutput=0
  wires:
  In/1 -> " "/1

== system simModel2020/AutoPilot/InnerLoopAutopilot/Longitudinal Channel经度通道/AutoThrottle/AT Mode = 0,Recycle/Filter1 ==
  x : Inport
  SW_x(k-1) : Inport  Port=2
  time : Inport  Port=3
  Constant : Constant  SampleTime=-1
  Data Type Conversion3 : DataTypeConversion  SaturateOnIntegerOverflow=off  RndMeth=Floor
  Detect Change : simulink/Logic and Bit Operations/Detect Change  vinit=0  OutDataTypeStr=boolean
  Gain : Gain  Gain=0.5
  Math Function : Math  SignedPower=on
  Product : Product
  Product1 : Product
  Subsystem : Subsystem
      mask Display: disp('S/H')
  Sum : Sum  Inputs=|+-
  Sum1 : Sum  Inputs=|++
  Sum2 : Sum  Inputs=+-|
  y : Outport
  wires:
  Product/1 -> Sum1/2
  SW_x(k-1)/1 -> Product/2
  Product1/1 -> Sum1/1
  x/1 -> Product1/1
  Sum1/1 -> Data Type Conversion3/1
  time/1 -> Subsystem/1(In), Sum2/2
  Subsystem/1(" ") -> Sum2/1
  Sum2/1 -> Gain/1
  Gain/1 -> Math Function/1
  Math Function/1 -> Sum/2, Product/1
  Sum/1 -> Product1/2
  Data Type Conversion3/1 -> y/1
  Constant/1 -> Detect Change/1, Sum/1
  Detect Change/1 -> Subsystem/Enable

== system simModel2020/AutoPilot/InnerLoopAutopilot/Longitudinal Channel经度通道/AutoThrottle/AT Mode = 0,Recycle/Rate Limiter Dynamic with External IC and Autoreset for Change in IC ==
  note: Y(k)
  note: U(k)
  up : Inport
  u : Inport  Port=2
  lo : Inport  Port=3
  IC : Inport  Port=4
  Abs : Abs  SaturateOnIntegerOverflow=off
  Delay : Delay  DelayLength=1
  Difference Inputs1 : Sum  Description=Add in CPU  DisableCoverage=on  Inputs=+-  OutDataTypeStr=Inherit: Inherit via back propagation
  Difference Inputs2 : Sum  Description=Add in CPU  OutDataTypeStr=Inherit: Inherit via back propagation
  Saturation Dynamic : Subsystem  mask(Saturation Dynamic){OutMin=[], OutMax=[], OutDataTypeStr=Inherit: Same as second input, OutputDataTypeScalingMode=Same as second input, OutDataType=fixdt(1, 16), OutScaling=2^-10, LockScale=off, RndMeth=Floor, DoSatur=off}
      mask prompts: OutMin "Simulink:masks:OutputMinimum_MP"; OutMax "Simulink:masks:OutputMaximum_MP"; OutDataTypeStr "Simulink:masks:OutputDataType_MP"; OutputDataTypeScalingMode "Simulink:masks:OutputDataTypeMode_MP"; OutDataType "Simulink:masks:OutputDataTypeegFixdt116Fixdtsingle_MP"; OutScaling "Simulink:masks:OutputScalingSlopeEg29OrSlopeBias_MP"; LockScale "Simulink:masks:LockOutputDataTypeAgainstFxpTools_MP"; RndMeth "Simulink:masks:IntegerRoundingMode_MP"; DoSatur "Simulink:masks:SaturateOnIntegerOverflow_MP"
      mask help: Simulink:masks:SaturationDynamic_MD
      mask init:
      | blkH = gcbh;
      | blkName = getfullname(blkH);
      | 
      | switch_blks = {'Switch','Switch2'}; 
      | for i = 1:length(switch_blks)
      |   set_param([blkName,'/',switch_blks{i}], ...
      |       'RndMeth', RndMeth, ...
      | 	  'DoSatur', DoSatur);
      | end
      | 
      | propBlk = [blkName, '/Data Type Propagation'];
      | 
      | if strcmp(OutputDataTypeScalingMode, 'Same as second input')
      |     set_param(propBlk, 'PropDataTypeMode', 'Inherit via propagation rule', ...
      |                        'PropScalingMode',  'Inherit via propagation rule');
      | else
      |     scaling = OutScaling;
      |     scalingMode = 'Specify via dialog';
      |     switch OutputDataTypeScalingMode
      |       case 'double'
      |         dataType = 'fixdt(''double'')';
      |       case 'single'
      |         dataType = 'fixdt(''single'')';
      |       case 'int8'
      |         dataType = 'fixdt(1,8,0)';
      |       case 'uint8'
      |         dataType = 'fixdt(0,8,0)';
      |       case 'int16'
      |         dataType = 'fixdt(1,16,0)';
      |       case 'uint16'
      |         dataType = 'fixdt(0,16,0)';
      |       case 'int32'
      |         dataType = 'fixdt(1,32,0)';
      |       case 'uint32'
      |         dataType = 'fixdt(0,32,0)';
      |       case 'Specify via dialog'
      |         dataType = OutDataType;
      |         if ~isempty(OutDataTypeStr) && isa(OutDataTypeStr,'Simulink.NumericType') 
      |           if strcmp(OutDataTypeStr.DataTypeMode, 'Fixed-point: unspecified scaling') 
      |             scalingMode = 'Obtain via best precision';
      |             range = [OutMin OutMax];
      |             range = range(~isinf(range));
      |             set_param(propBlk, 'ValuesUsedBestPrec', mat2str(range));
      |           end
      |         end
      |     end
      |     
      |     set_param(propBlk, 'PropDataTypeMode', 'Specify via dialog', ...
      |                        'PropScalingMode',  scalingMode, ...
      |                        'PropDataType',     dataType, ...
      |                        'PropScaling',      scaling);
      | end
      mask Callback OutDataTypeStr: fixptdialog(gcbh)
      mask TypeOptions OutputDataTypeScalingMode: double | single | int8 | uint8 | int16 | uint16 | int32 | uint32 | Specify via dialog | Same as second input
      mask Callback OutputDataTypeScalingMode: fixptdialog(gcbh)
      mask Callback OutDataType: fixptdialog(gcbh)
      mask TypeOptions RndMeth: Simulink:masks:Ceiling | Simulink:masks:Convergent | Simulink:masks:Floor | Simulink:masks:Nearest | Simulink:masks:Round | Simulink:masks:Simplest | Simulink:masks:Zero
  Subsystem : Subsystem
  Subtract : Sum  Inputs=+-
  Unit Delay Resettable External IC : Subsystem  mask(Unit Delay Resettable External Initial Condition){tsamp=-1}
      mask prompts: tsamp "Simulink:masks:SampleTime_MP"
      mask help: Simulink:masks:UnitDelayResettableExternalInitialCondition_MD
      mask Display: dpoly(1,[1 0],'z')
  delta fall limit : Product  DisableCoverage=on  Inputs=**  OutDataTypeStr=Inherit: Inherit via back propagation  SaturateOnIntegerOverflow=on
  delta rise limit : Product  DisableCoverage=on  Inputs=**  OutDataTypeStr=Inherit: Inherit via back propagation  SaturateOnIntegerOverflow=on
  sample time : SampleTimeMath  DisableCoverage=on  TsampMathOp=Ts Only  weightValue=1
  Y : Outport
  wires:
  Abs/1 -> Subsystem/1(WP Fly)
  Subsystem/1(Just Enab) -> Unit Delay Resettable External IC/2(R)
  Subtract/1 -> Abs/1
  Delay/1 -> Subtract/1
  sample time/1 -> delta fall limit/2, delta rise limit/2
  lo/1 -> delta fall limit/1
  delta rise limit/1 -> Saturation Dynamic/1(up)
  up/1 -> delta rise limit/1
  Difference Inputs2/1 -> Unit Delay Resettable External IC/1(u), Y/1
  Unit Delay Resettable External IC/1(y) -> Difference Inputs1/2, Difference Inputs2/2  "Y(k-1)"
  Saturation Dynamic/1(y) -> Difference Inputs2/1
  delta fall limit/1 -> Saturation Dynamic/3(lo)
  u/1 -> Difference Inputs1/1, sample time/1
  Difference Inputs1/1 -> Saturation Dynamic/2(u)  "( U(k) - Y(k-1) )"
  IC/1 -> Delay/1, Unit Delay Resettable External IC/3(IC), Subtract/2

== system simModel2020/AutoPilot/InnerLoopAutopilot/Longitudinal Channel经度通道/AutoThrottle/AT Mode = 2,MCP Speed/Filter1 ==
  x : Inport
  SW_x(k-1) : Inport  Port=2
  time : Inport  Port=3
  Constant : Constant  SampleTime=-1
  Data Type Conversion3 : DataTypeConversion  SaturateOnIntegerOverflow=off  RndMeth=Floor
  Detect Change : simulink/Logic and Bit Operations/Detect Change  vinit=0  OutDataTypeStr=boolean
  Gain : Gain  Gain=0.05
  Math Function : Math  SignedPower=on
  Product : Product
  Product1 : Product
  Subsystem : Subsystem
      mask Display: disp('S/H')
  Sum : Sum  Inputs=|+-
  Sum1 : Sum  Inputs=|++
  Sum2 : Sum  Inputs=+-|
  y : Outport
  wires:
  Product/1 -> Sum1/2
  SW_x(k-1)/1 -> Product/2
  Product1/1 -> Sum1/1
  x/1 -> Product1/1
  Sum1/1 -> Data Type Conversion3/1
  time/1 -> Subsystem/1(In), Sum2/2
  Subsystem/1(" ") -> Sum2/1
  Sum2/1 -> Gain/1
  Gain/1 -> Math Function/1
  Math Function/1 -> Sum/2, Product/1
  Sum/1 -> Product1/2
  Data Type Conversion3/1 -> y/1
  Constant/1 -> Detect Change/1, Sum/1
  Detect Change/1 -> Subsystem/Enable

== system simModel2020/AutoPilot/InnerLoopAutopilot/Longitudinal Channel经度通道/AutoThrottle/AT Mode = 2,MCP Speed/N1_Control ==
  N1_Cmd : Inport
  N1 : Inport  Port=2
  Add1 : Sum  Inputs=+-
  Derivative1 : Derivative
  Gain3 : Gain  Gain=0.1
  Gain4 : Gain  Gain=0.02
  Integrator1 : Integrator  LimitOutput=on  UpperSaturationLimit=1  LowerSaturationLimit=0
  Sum1 : Sum  Inputs=++|
  Throttle Limit3 : Saturate  UpperLimit=0.2  LowerLimit=-0.2
      settings: AttributesFormatString="[%<LowerLimit>  %<UpperLimit>]"
  dT : Outport
  wires:
  Gain4/1 -> Sum1/1
  Integrator1/1 -> dT/1
  Gain3/1 -> Sum1/2
  Sum1/1 -> Throttle Limit3/1
  Throttle Limit3/1 -> Integrator1/1
  N1_Cmd/1 -> Add1/1
  Add1/1 -> Derivative1/1, Gain3/1
  Derivative1/1 -> Gain4/1
  N1/1 -> Add1/2

== system simModel2020/AutoPilot/InnerLoopAutopilot/Longitudinal Channel经度通道/AutoThrottle/AT Mode = 2,MCP Speed/sat_integration ==
  err : Inport
  Constant1 : Constant  Value=10
  Constant2 : Constant  Value=0
  Gain2 : Gain  Gain=0.5
  Integrator : Integrator  LimitOutput=on  UpperSaturationLimit=220  LowerSaturationLimit=0
  Interval Test Dynamic : simulink/Logic and Bit Operations/Interval Test Dynamic  IntervalClosedRight=on  IntervalClosedLeft=on  OutDataTypeStr=boolean
  Switch : Switch  Criteria=u2 > Threshold  Threshold=0.5  SaturateOnIntegerOverflow=off  InputSameDT=off
  Unary Minus : UnaryMinus
  int_err : Outport
  wires:
  err/1 -> Interval Test Dynamic/2, Switch/1
  Constant1/1 -> Interval Test Dynamic/1, Unary Minus/1
  Gain2/1 -> int_err/1
  Constant2/1 -> Switch/3
  Interval Test Dynamic/1 -> Switch/2
  Unary Minus/1 -> Interval Test Dynamic/3
  Integrator/1 -> Gain2/1
  Switch/1 -> Integrator/1
